simulink model "readacc_16bit"  (R2017b)
settings: Solver=VariableStepAuto  StartTime=0.0  StopTime=15  RelTol=1e-3
libraries: instrumentlib x1
settings Model: Creator=jmd  LastModifiedBy=jmd

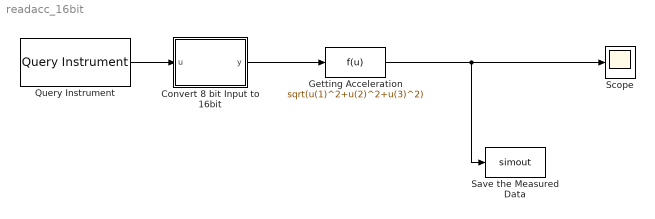
== system readacc_16bit ==
  Convert 8 bit Input to 16bit : MATLAB Function  TreatAsAtomicUnit=on
  Getting Acceleration : Fcn  Expr=sqrt(u(1)^2+u(2)^2+u(3)^2)
  Query Instrument : instrumentlib/Query Instrument  sampleTime=0.003  isWorkspaceObject=off  timeout=10  inputBufferSize=512  protocol=Serial  serialPort=COM1  baudRate=57600  gpibVendor=Agilent Technologies  boardIndex=0  primaryAddress=1  secondaryAddress=0  visaVendor=Agilent  visaSerialPort=0  chassisIndex=0  logicalAddress=0  tcpRemoteHost='127.0.0.1'  tcpRemotePort=4500  udpRemoteHost='127.0.0.1'  udpRemotePort=9090  visaTCPBoardIndex=0  visaTCPRemoteHost='127.0.0.1'  usbBoardIndex=0  usbManufID=0  usbModelCode=0  usbSerialNumber=0  initAction=None  initCommand='DATA:SOURCE CH1'  initFunction=get  queryCommand=''  responseFormat=Binary  asciiFormatting='%d,'  precision=8-bit integer  byteOrder=Little endian  valuesToRead=1  removeBytes=off  afterOutputAction=Repeat query for new data  enableFrames=on  frameSize=7
      settings: SourceProductName=Instrument Control Toolbox  SourceProductBaseCode=IC
  Save the Measured Data : ToWorkspace  VariableName=simout  SaveFormat=Timeseries  SampleTime=-1
  Scope : Scope
  wires:
  Getting Acceleration/1 -> Save the Measured Data/1, Scope/1
  Query Instrument/1 -> Convert 8 bit Input to 16bit/1(u)
  Convert 8 bit Input to 16bit/1(y) -> Getting Acceleration/1

== matlab function readacc_16bit/Convert 8 bit Input to 16bit ==
  data: u input; y output
function y = fcn(u)
u2 = zeros(7,1);
for i = 1:7
    if u(i) == -127
        u2=[u((i+1):7);u(1:i)];
        break
    end
end
y1 = u2(1)*256+u2(2);
y2 = u2(3)*256+u2(4);
y3 = u2(5)*256+u2(6);
y=[y1,y2,y3];
